simulink model "TakagiSugenaConControl1"  (R2025a)
settings: Solver=FixedStepAuto  StartTime=0.0  StopTime=5  FixedStep=.001  RelTol=1e-3
values from neighbouring files (symbols this model uses):
  K_nl = place(A1, B1, p)    [KnlKnsKz.m]    (also in linealizar_TS_regulador.m = K_nl(:).')
  K_ns = place(A2, B2, p)    [KnlKnsKz.m]    (also in linealizar_TS_regulador.m = K_ns(:).')
  K_z = place(A3, B3, p)    [KnlKnsKz.m]    (also in linealizar_TS_regulador.m = K_z(:).')
undefined symbols (not defined in the file or in its folder): G_nl, G_ns, G_z, P_nl, P_ns, P_z
settings Model: Creator=aceve  LastModifiedBy=aceve

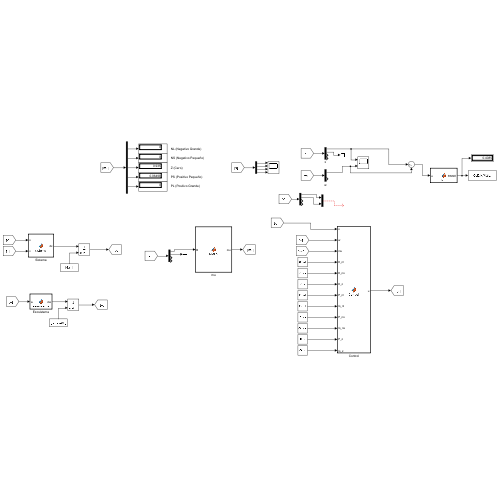
[thumbnail: Simulink's stored preview of the top-level diagram]
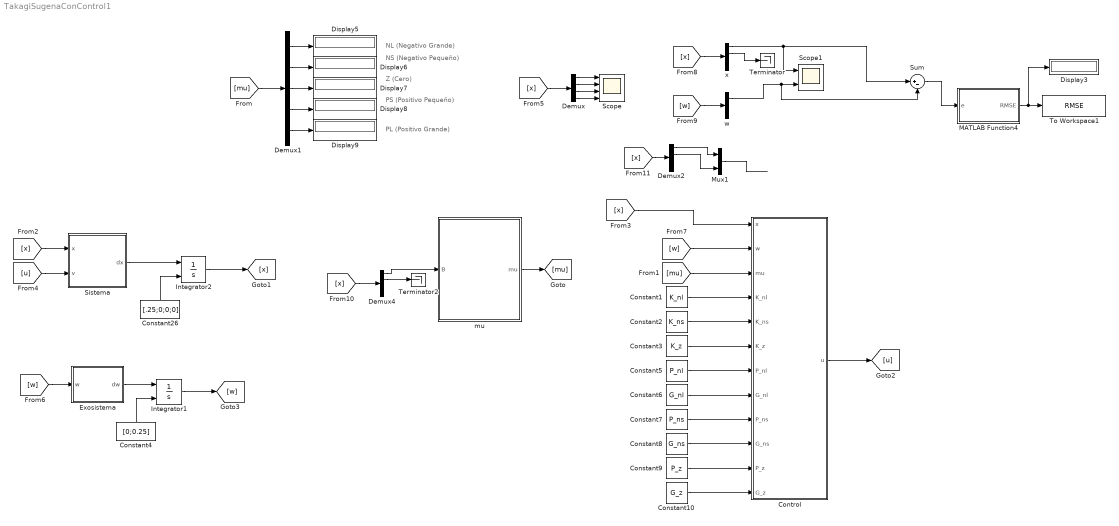
== system TakagiSugenaConControl1 ==
  note: PS (Positivo Pequeño)
  note: NL (Negativo Grande)
  note: NS (Negativo Pequeño)
  note: PL (Positivo Grande)
  note: Z (Cero)
  Constant1 : Constant  Value=K_nl
  Constant10 : Constant  Value=G_z
  Constant2 : Constant  Value=K_ns
  Constant26 : Constant  Value=[.25;0;0;0]
  Constant3 : Constant  Value=K_z
  Constant4 : Constant  Value=[0;0.25]
  Constant5 : Constant  Value=P_nl
  Constant6 : Constant  Value=G_nl
  Constant7 : Constant  Value=P_ns
  Constant8 : Constant  Value=G_ns
  Constant9 : Constant  Value=P_z
  Control : MATLAB Function  TreatAsAtomicUnit=on
  Demux : Demux
  Demux1 : Demux  Outputs=5
  Demux2 : Demux
  Demux4 : Demux
  Display{3,5..9} (6 alike) : Display
  Exosistema : MATLAB Function  TreatAsAtomicUnit=on
  Integrator1 : Integrator  InitialConditionSource=external
  Integrator2 : Integrator  InitialConditionSource=external
  MATLAB Function4 : MATLAB Function  TreatAsAtomicUnit=on
  Mux1 : Mux  Inputs=2
  Scope : Scope  NumInputPorts=4
      settings: ActiveDisplayYMinimum=-3.2104722777613426  ActiveDisplayYMaximum=3.2104673095886191
  Scope1 : Scope  NumInputPorts=2
      settings: ActiveDisplayYMinimum=-0.704911395213558  ActiveDisplayYMaximum=0.75289038131529185
  Sistema : MATLAB Function  TreatAsAtomicUnit=on
  Sum : Sum  Inputs=|+-
  Terminator : Terminator
  Terminator2 : Terminator
  To Workspace1 : ToWorkspace  VariableName=RMSE  SaveFormat=Structure With Time  SampleTime=-1
  mu : MATLAB Function  TreatAsAtomicUnit=on
  w : Demux  Outputs=2
  x : Demux
  wires:
  mu/1(mu) -> [mu]
  Demux1/1 -> Display5/1
  Demux1/4 -> Display8/1
  Demux1/5 -> Display9/1
  Demux1/2 -> Display6/1
  Demux1/3 -> Display7/1
  [mu] -> Demux1/1
  [mu] -> Control/3(mu)
  Control/1(u) -> [u]
  [x] -> Demux/1
  Demux/1 -> Scope/1
  Demux/2 -> Scope/2
  Constant1/1 -> Control/4(K_nl)
  Constant2/1 -> Control/5(K_ns)
  Constant3/1 -> Control/6(K_z)
  Constant4/1 -> Integrator1/2
  Exosistema/1(dw) -> Integrator1/1
  Integrator1/1 -> [w]
  [w] -> Exosistema/1(w)
  [w] -> Control/2(w)
  x/1 -> Sum/1, Scope1/1
  [x] -> x/1
  x/2 -> Terminator/1
  [w] -> w/1
  [x] -> Demux4/1
  Demux4/1 -> mu/1(B)
  Demux4/2 -> Terminator2/1
  Constant5/1 -> Control/7(P_nl)
  Constant6/1 -> Control/8(G_nl)
  Constant7/1 -> Control/9(P_ns)
  Constant8/1 -> Control/10(G_ns)
  Constant9/1 -> Control/11(P_z)
  Constant10/1 -> Control/12(G_z)
  Constant26/1 -> Integrator2/2
  [x] -> Sistema/1(x)
  Sistema/1(dx) -> Integrator2/1
  Integrator2/1 -> [x]
  Demux/3 -> Scope/3
  Demux/4 -> Scope/4
  [u] -> Sistema/2(v)
  Demux2/1 -> Mux1/1
  Mux1/1 -> ?
  [x] -> Demux2/1
  Demux2/2 -> Mux1/2
  [x] -> Control/1(x)
  MATLAB Function4/1(RMSE) -> Display3/1, To Workspace1/1
  Sum/1 -> MATLAB Function4/1(e)
  w/1 -> Sum/2, Scope1/2

== matlab function TakagiSugenaConControl1/Control ==
  data: x input; u output; w input; mu input; K_nl input; K_ns input; K_z input; P_nl input; G_nl input; P_ns input; G_ns input; P_z input; G_z input
function u = Control(x, w, mu, K_nl, K_ns, K_z, P_nl, G_nl, P_ns, G_ns, P_z, G_z)
% x  : estados [theta; dtheta; x_carro; dx_carro] (4x1)
% w  : exosistema [w1; w2] (2x1)
% mu : vector de membresías [NL NS Z PS PL]
% K_*: ganancias (1x4)
% P_*: matrices de Francis (4x2)
% G_*: matrices de Francis (1x2)

% Asegurar formato fila
K_nl = K_nl(:).';  G_nl = G_nl(:).';
K_ns = K_ns(:).';  G_ns = G_ns(:).';
K_z  = K_z(:).';   G_z  = G_z(:).';

% --- Región NL / PL ---
% NO recortar K, se usa completo (1x4)
u_nl = -K_nl*x + (G_nl - K_nl*P_nl)*w;   % escalar
u_pl = u_nl;

% --- Región NS / PS ---
u_ns = -K_ns*x + (G_ns - K_ns*P_ns)*w;
u_ps = u_ns;

% --- Región Z ---
u_z = -K_z*x + (G_z - K_z*P_z)*w;

% --- Defuzzificación ---
num = mu(1)*u_nl + mu(2)*u_ns + mu(3)*u_z + mu(4)*u_ps + mu(5)*u_pl;
den = sum(mu) + 1e-12;  % evitar división por cero
u   = num/den;
end

== matlab function TakagiSugenaConControl1/mu ==
  data: B input; mu output
function mu = triMF5(B)
% mu = [NL NS Z PS PL]
mu = zeros(5,1);
% breakpoints
n15 = -15; n7 = -7.5; z0 = 0; p7 = 7.5; p15 = 15;

% NL
if B <= n15
    mu(1) = 1;
elseif B <= n7
    mu(1) = (n7 - B)/7.5;
else
    mu(1) = 0;
end

% NS
if B <= n15
    mu(2) = 0;
elseif B <= n7
    mu(2) = (B - n15)/7.5;
elseif B <= z0
    mu(2) = (z0 - B)/7.5;
else
    mu(2) = 0;
end

% Z
if B <= n7
    mu(3) = 0;
elseif B <= z0
    mu(3) = (B - n7)/7.5;
elseif B <= p7
    mu(3) = (p7 - B)/7.5;
else
    mu(3) = 0;
end

% PS
if B <= z0
    mu(4) = 0;
elseif B <= p7
    mu(4) = (B - z0)/7.5;
elseif B <= p15
    mu(4) = (p15 - B)/7.5;
else
    mu(4) = 0;
end

% PL
if B <= p7
    mu(5) = 0;
elseif B < p15
    mu(5) = (B - p7)/7.5;
else
    mu(5) = 1;
end

== matlab function TakagiSugenaConControl1/Exosistema ==
  data: w input; dw output
function dw = exosistema(w)

dw = [0 10; -10 0]*w;

== matlab function TakagiSugenaConControl1/Sistema ==
  data: x input; dx output; v input
function dx = sistema(x, v)


dx = zeros(4,1);   % asegura tamaño fijo 4x1

M = 0.5;     % (M) Masa del carro (kg)
m = 0.2;     % (m) Masa del péndulo (kg)
l = 0.3;     % (l) Longitud del péndulo (m)
g = 9.81;    % (g) Gravedad (m/s^2)

th     = x(1);    % x1: ángulo péndulo
dth    = x(2);    % x2: velocidad angular péndulo
x_pos  = x(3);    % x3: posición carro
dx_pos = x(4);    % x4: velocidad carro


F_input = v(1);

s_th = sin(th);
c_th = cos(th);

% Denominador común
den_common = (m * s_th^2 + M);

% Calcular ddth (x2_dot)
num_x2 = F_input*c_th + (M+m)*g*s_th - m*l*dth^2*s_th*c_th;
den_x2 = den_common * l;
ddth = num_x2 / den_x2;

% Calcular ddx_pos (x4_dot)
num_x4 = F_input + m*g*s_th*c_th - m*l*dth^2*s_th;
den_x4 = den_common;
ddx_pos = num_x4 / den_x4;

%% ---- Derivadas de estado ----
dx(1) = dth;
dx(2) = ddth;
dx(3) = dx_pos;
dx(4) = ddx_pos;

end

== matlab function TakagiSugenaConControl1/MATLAB Function4 ==
  settings: updateMethod=DISCRETE
  data: e input; RMSE output
function RMSE = fcn(e)
% e: error escalar (por ejemplo, error_pitch o error_yaw)
% RMSE: raíz del error cuadrático medio acumulada (escalar)

persistent S_E2 N
if isempty(S_E2)
    S_E2 = 0;
    N    = uint32(0);
end

e    = double(e);   % asegura tipo
S_E2 = S_E2 + e.^2; % acumula e^2
N    = N + 1;       % cuenta muestras

RMSE = sqrt( S_E2 / max(1,double(N)) );
end
